simulink model "odsprzeganie"  (R2017a)
settings: Solver=FixedStepAuto  StartTime=0.0  StopTime=6000  RelTol=1e-3
values from neighbouring files (symbols this model uses):
  a = 8    [TAP_Projekt1.m]    (also in ZNExperiment.m; decoupling.m; matlab.mat; regInit.m)
  C = [0 1; 1 0]    [TAP_Projekt1.m]    (also in ZNExperiment.m = 0.4; decoupling.m = 0.4; matlab.mat = [1  0; 0  1]; regInit.m = 0.4)
  TCp = 21    [TAP_Projekt1.m]    (also in ZNExperiment.m; decoupling.m; matlab.mat; regInit.m)
  TDp = 30    [TAP_Projekt1.m]    (also in ZNExperiment.m; decoupling.m; matlab.mat; regInit.m)
  THp = 64    [TAP_Projekt1.m]    (also in ZNExperiment.m; decoupling.m; matlab.mat; regInit.m)
undefined symbols (not defined in the file or in its folder): teta, tetaC
libraries: simulink x4, cstblocks x2
settings Model: Creator=Barteux  LastModifiedBy=Barteux

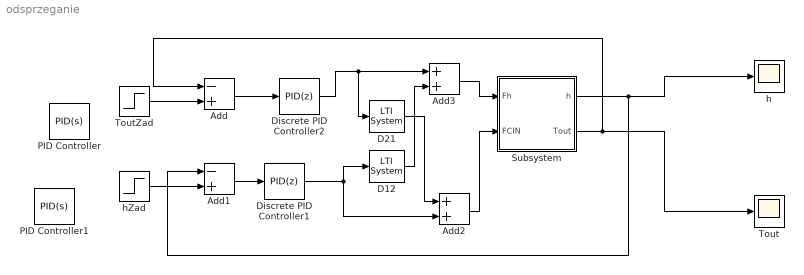
== system odsprzeganie ==
  Add : Sum  Inputs=-+
  Add1 : Sum  Inputs=-+
  Add2 : Sum
  Add3 : Sum
  D12 : cstblocks/LTI System  sys=D12_z  IC=[]
  D21 : cstblocks/LTI System  sys=D21_z  IC=[]
  Discrete PID Controller1 : simulink/Continuous/PID Controller  Controller=PID  TimeDomain=Discrete-time  SampleTime=1  IntegratorMethod=Forward Euler  FilterMethod=Forward Euler  Form=Parallel  UseFilter=on  ControllerParametersSource=internal  P=0.180678962603669  I=0.00106729417698503  D=0  N=100  InitialConditionSource=internal  InitialConditionForIntegrator=0  InitialConditionForFilter=0  ExternalReset=none  LimitOutput=off  UpperSaturationLimit=inf  LowerSaturationLimit=-inf  LinearizeAsGain=off  AntiWindupMode=none  Kb=1  TrackingMode=off  Kt=1  PParamMin=[]  PParamMax=[]  IParamMin=[]  IParamMax=[]  DParamMin=[]  DParamMax=[]  NParamMin=[]  NParamMax=[]  KbParamMin=[]  KbParamMax=[]  KtParamMin=[]  KtParamMax=[]  POutMin=[]  POutMax=[]  IOutMin=[]  IOutMax=[]  DOutMin=[]  DOutMax=[]  NOutMin=[]  NOutMax=[]  KbOutMin=[]  KbOutMax=[]  KtOutMin=[]  KtOutMax=[]  IntegratorOutMin=[]  IntegratorOutMax=[]  FilterOutMin=[]  FilterOutMax=[]  SumOutMin=[]  SumOutMax=[]  SumI1OutMin=[]  SumI1OutMax=[]  SumI2OutMin=[]  SumI2OutMax=[]  SumI3OutMin=[]  SumI3OutMax=[]  SumDOutMin=[]  SumDOutMax=[]  SaturationOutMin=[]  SaturationOutMax=[]  IntegratorContinuousStateAttributes=''  IntegratorStateMustResolveToSignalObject=off  IntegratorRTWStateStorageClass=Auto  FilterContinuousStateAttributes=''  FilterStateMustResolveToSignalObject=off  FilterRTWStateStorageClass=Auto  DifferentiatorICPrevScaledInput=0  DifferentiatorOutMin=[]  DifferentiatorOutMax=[]  InitialConditionSetting=State (most efficient)
  Discrete PID Controller2 : simulink/Continuous/PID Controller  Controller=PID  TimeDomain=Discrete-time  SampleTime=1  IntegratorMethod=Forward Euler  FilterMethod=Forward Euler  Form=Parallel  UseFilter=on  ControllerParametersSource=internal  P=0.600392409469819  I=0.0259650078715821  D=0  N=100  InitialConditionSource=internal  InitialConditionForIntegrator=0  InitialConditionForFilter=0  ExternalReset=none  LimitOutput=off  UpperSaturationLimit=inf  LowerSaturationLimit=-inf  LinearizeAsGain=off  AntiWindupMode=none  Kb=1  TrackingMode=off  Kt=1  PParamMin=[]  PParamMax=[]  IParamMin=[]  IParamMax=[]  DParamMin=[]  DParamMax=[]  NParamMin=[]  NParamMax=[]  KbParamMin=[]  KbParamMax=[]  KtParamMin=[]  KtParamMax=[]  POutMin=[]  POutMax=[]  IOutMin=[]  IOutMax=[]  DOutMin=[]  DOutMax=[]  NOutMin=[]  NOutMax=[]  KbOutMin=[]  KbOutMax=[]  KtOutMin=[]  KtOutMax=[]  IntegratorOutMin=[]  IntegratorOutMax=[]  FilterOutMin=[]  FilterOutMax=[]  SumOutMin=[]  SumOutMax=[]  SumI1OutMin=[]  SumI1OutMax=[]  SumI2OutMin=[]  SumI2OutMax=[]  SumI3OutMin=[]  SumI3OutMax=[]  SumDOutMin=[]  SumDOutMax=[]  SaturationOutMin=[]  SaturationOutMax=[]  IntegratorContinuousStateAttributes=''  IntegratorStateMustResolveToSignalObject=off  IntegratorRTWStateStorageClass=Auto  FilterContinuousStateAttributes=''  FilterStateMustResolveToSignalObject=off  FilterRTWStateStorageClass=Auto  DifferentiatorICPrevScaledInput=0  DifferentiatorOutMin=[]  DifferentiatorOutMax=[]  InitialConditionSetting=State (most efficient)
  PID Controller : simulink/Continuous/PID Controller  Controller=PID  TimeDomain=Continuous-time  SampleTime=-1  IntegratorMethod=Forward Euler  FilterMethod=Forward Euler  Form=Parallel  UseFilter=on  ControllerParametersSource=internal  P=0.000829547017946  I=0.024693739630127  D=0  N=100  InitialConditionSource=internal  InitialConditionForIntegrator=0  InitialConditionForFilter=0  ExternalReset=none  LimitOutput=off  UpperSaturationLimit=inf  LowerSaturationLimit=-inf  LinearizeAsGain=on  AntiWindupMode=none  Kb=1  TrackingMode=off  Kt=1  PParamMin=[]  PParamMax=[]  IParamMin=[]  IParamMax=[]  DParamMin=[]  DParamMax=[]  NParamMin=[]  NParamMax=[]  KbParamMin=[]  KbParamMax=[]  KtParamMin=[]  KtParamMax=[]  POutMin=[]  POutMax=[]  IOutMin=[]  IOutMax=[]  DOutMin=[]  DOutMax=[]  NOutMin=[]  NOutMax=[]  KbOutMin=[]  KbOutMax=[]  KtOutMin=[]  KtOutMax=[]  IntegratorOutMin=[]  IntegratorOutMax=[]  FilterOutMin=[]  FilterOutMax=[]  SumOutMin=[]  SumOutMax=[]  SumI1OutMin=[]  SumI1OutMax=[]  SumI2OutMin=[]  SumI2OutMax=[]  SumI3OutMin=[]  SumI3OutMax=[]  SumDOutMin=[]  SumDOutMax=[]  SaturationOutMin=[]  SaturationOutMax=[]  IntegratorContinuousStateAttributes=''  IntegratorStateMustResolveToSignalObject=off  IntegratorRTWStateStorageClass=Auto  FilterContinuousStateAttributes=''  FilterStateMustResolveToSignalObject=off  FilterRTWStateStorageClass=Auto  DifferentiatorICPrevScaledInput=0  DifferentiatorOutMin=[]  DifferentiatorOutMax=[]  InitialConditionSetting=State (most efficient)
  PID Controller1 : simulink/Continuous/PID Controller  Controller=PID  TimeDomain=Continuous-time  SampleTime=-1  IntegratorMethod=Forward Euler  FilterMethod=Forward Euler  Form=Parallel  UseFilter=on  ControllerParametersSource=internal  P=0.10337475454881  I=0.00070325675501345  D=0  N=100  InitialConditionSource=internal  InitialConditionForIntegrator=0  InitialConditionForFilter=0  ExternalReset=none  LimitOutput=off  UpperSaturationLimit=inf  LowerSaturationLimit=-inf  LinearizeAsGain=on  AntiWindupMode=none  Kb=1  TrackingMode=off  Kt=1  PParamMin=[]  PParamMax=[]  IParamMin=[]  IParamMax=[]  DParamMin=[]  DParamMax=[]  NParamMin=[]  NParamMax=[]  KbParamMin=[]  KbParamMax=[]  KtParamMin=[]  KtParamMax=[]  POutMin=[]  POutMax=[]  IOutMin=[]  IOutMax=[]  DOutMin=[]  DOutMax=[]  NOutMin=[]  NOutMax=[]  KbOutMin=[]  KbOutMax=[]  KtOutMin=[]  KtOutMax=[]  IntegratorOutMin=[]  IntegratorOutMax=[]  FilterOutMin=[]  FilterOutMax=[]  SumOutMin=[]  SumOutMax=[]  SumI1OutMin=[]  SumI1OutMax=[]  SumI2OutMin=[]  SumI2OutMax=[]  SumI3OutMin=[]  SumI3OutMax=[]  SumDOutMin=[]  SumDOutMax=[]  SaturationOutMin=[]  SaturationOutMax=[]  IntegratorContinuousStateAttributes=''  IntegratorStateMustResolveToSignalObject=off  IntegratorRTWStateStorageClass=Auto  FilterContinuousStateAttributes=''  FilterStateMustResolveToSignalObject=off  FilterRTWStateStorageClass=Auto  DifferentiatorICPrevScaledInput=0  DifferentiatorOutMin=[]  DifferentiatorOutMax=[]  InitialConditionSetting=State (most efficient)
  Subsystem : Subsystem
  Tout : Scope
  ToutZad : Step  Time=1600  Before=36  After=36  SampleTime=0
  h : Scope
  hZad : Step  Time=3500  Before=58  After=65  SampleTime=0
  wires:
  Subsystem/1(h) -> Add1/1, h/1
  Subsystem/2(Tout) -> Add/1, Tout/1
  ToutZad/1 -> Add/2
  Discrete PID Controller2/1 -> D21/1, Add3/1
  hZad/1 -> Add1/2
  Add1/1 -> Discrete PID Controller1/1
  Add/1 -> Discrete PID Controller2/1
  Discrete PID Controller1/1 -> D12/1, Add2/2
  Add2/1 -> Subsystem/2(FCIN)
  Add3/1 -> Subsystem/1(Fh)
  D21/1 -> Add2/1
  D12/1 -> Add3/2

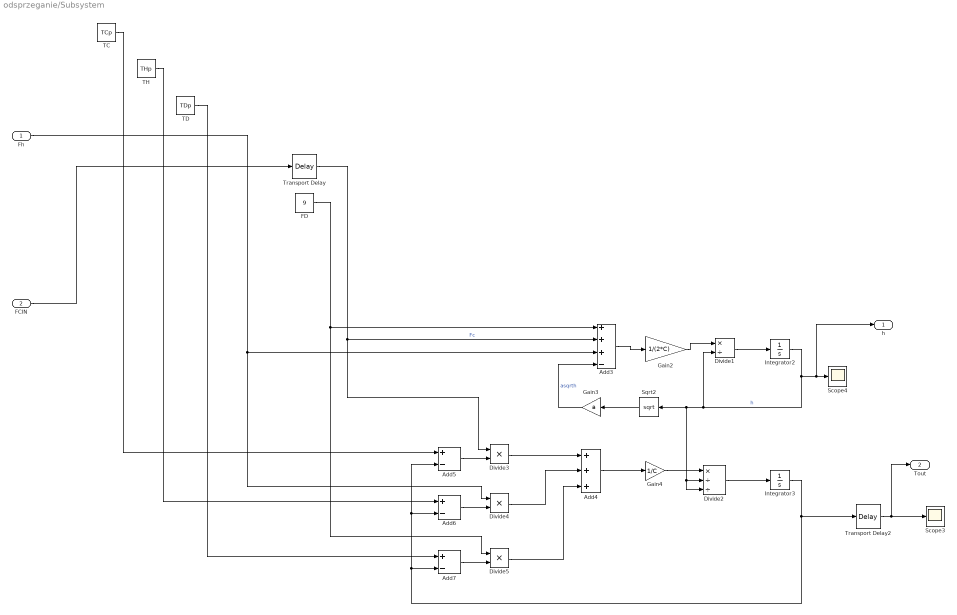
== system odsprzeganie/Subsystem ==
  Fh : Inport
  FCIN : Inport  Port=2
  Add3 : Sum  Inputs=+++-
  Add4 : Sum  Inputs=+++
  Add5 : Sum  Inputs=+-
  Add6 : Sum  Inputs=+-
  Add7 : Sum  Inputs=+-
  Divide1 : Product  Inputs=*/
  Divide2 : Product  Inputs=*//
  Divide3 : Product  Inputs=**
  Divide4 : Product  Inputs=**
  Divide5 : Product  Inputs=**
  FD : Constant  Value=9
  Gain2 : Gain  Gain=1/(2*C)
  Gain3 : Gain  Gain=a
  Gain4 : Gain  Gain=1/C
  Integrator2 : Integrator  InitialCondition=54
  Integrator3 : Integrator  InitialCondition=30
  Scope3 : Scope
  Scope4 : Scope
  Sqrt2 : Sqrt  OutputSignalType=real  SaturateOnIntegerOverflow=on
  TC : Constant  Value=TCp
  TD : Constant  Value=TDp
  TH : Constant  Value=THp
  Transport Delay : TransportDelay  DelayTime=tetaC
  Transport Delay2 : TransportDelay  DelayTime=teta
  h : Outport
  Tout : Outport  Port=2
  wires:
  Fh/1 -> Divide4/1, Add3/3
  TD/1 -> Add7/1
  TH/1 -> Add6/1
  Transport Delay/1 -> Divide3/1, Add3/2  "Fc"
  FD/1 -> Divide5/1, Add3/1
  Integrator2/1 -> h/1, Scope4/1, Divide2/3, Divide2/2, Sqrt2/1, Divide1/2  "h"
  Add5/1 -> Divide3/2
  Sqrt2/1 -> Gain3/1
  Gain4/1 -> Divide2/1
  Divide1/1 -> Integrator2/1
  Add3/1 -> Gain2/1
  Divide2/1 -> Integrator3/1
  Add6/1 -> Divide4/2
  Add4/1 -> Gain4/1
  Gain2/1 -> Divide1/1
  Transport Delay2/1 -> Tout/1, Scope3/1
  Gain3/1 -> Add3/4  "asqrth"
  Divide5/1 -> Add4/3
  TC/1 -> Add5/1
  Integrator3/1 -> Add7/2, Add6/2, Add5/2, Transport Delay2/1
  Divide3/1 -> Add4/1
  Add7/1 -> Divide5/2
  Divide4/1 -> Add4/2
  FCIN/1 -> Transport Delay/1
